simulink model "Sim"  (R2019b)
settings: Solver=VariableStepAuto  StartTime=0.0  StopTime=10.0  RelTol=1e-3
undefined symbols (not defined in the file): damping, DiscIntNeverNeededParam, Id0, inertia, initial_percentage, Iq0, J, K_damping, K_inertia, L_ap, L_inc, L_inc_inv, Ldd_inc, Ldq_inc, Lqq_inc, Psi_dm, Qp, Qx, R, Rs, Tob, Tsim, Ud0, Umd, Umq, Uq0, we0, weh
settings Model: SimulationMode=accelerator  Creator=Downstream  LastModifiedBy=Downstream

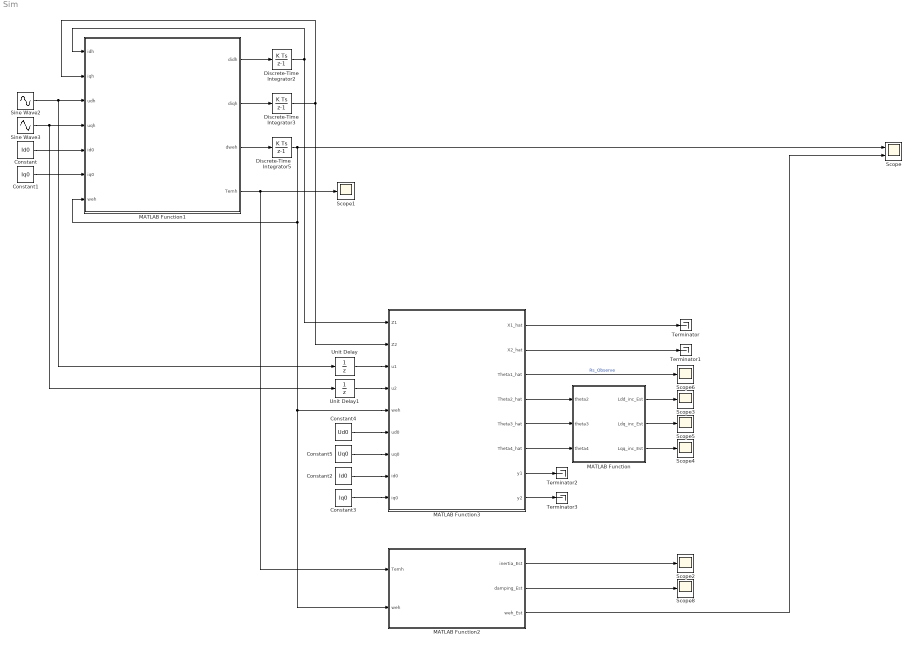
== system Sim ==
  Constant : Constant  Value=Id0  SampleTime=-1
  Constant1 : Constant  Value=Iq0  SampleTime=-1
  Constant2 : Constant  Value=Id0  SampleTime=-1
  Constant3 : Constant  Value=Iq0  SampleTime=-1
  Constant4 : Constant  Value=Ud0  SampleTime=-1
  Constant5 : Constant  Value=Uq0  SampleTime=-1
  Discrete-Time Integrator2 : DiscreteIntegrator  SampleTime=Tsim  ICPrevOutput=DiscIntNeverNeededParam  ICPrevScaledInput=DiscIntNeverNeededParam
  Discrete-Time Integrator3 : DiscreteIntegrator  SampleTime=Tsim  ICPrevOutput=DiscIntNeverNeededParam  ICPrevScaledInput=DiscIntNeverNeededParam
  Discrete-Time Integrator5 : DiscreteIntegrator  SampleTime=Tsim  ICPrevOutput=DiscIntNeverNeededParam  ICPrevScaledInput=DiscIntNeverNeededParam
  MATLAB Function : MATLAB Function  TreatAsAtomicUnit=on
  MATLAB Function1 : MATLAB Function  TreatAsAtomicUnit=on
  MATLAB Function2 : MATLAB Function  TreatAsAtomicUnit=on  SystemSampleTime=Tob
  MATLAB Function3 : MATLAB Function  TreatAsAtomicUnit=on  SystemSampleTime=Tob
  Scope : Scope  NumInputPorts=2
  Scope{1..6,8} (7 alike) : Scope
  Sine Wave2 : Sin  Amplitude=Umd  Frequency=weh  SampleTime=Tsim
  Sine Wave3 : Sin  Amplitude=Umq  Frequency=weh  Phase=pi/2  SampleTime=Tsim
  Terminator{,1..3} (4 alike) : Terminator
  Unit Delay : UnitDelay  SampleTime=Tob  HasFrameUpgradeWarning=on
  Unit Delay1 : UnitDelay  SampleTime=Tob  HasFrameUpgradeWarning=on
  wires:
  MATLAB Function1/1(didh) -> Discrete-Time Integrator2/1
  MATLAB Function1/2(diqh) -> Discrete-Time Integrator3/1
  Constant/1 -> MATLAB Function1/5(id0)
  Constant1/1 -> MATLAB Function1/6(iq0)
  MATLAB Function1/3(dweh) -> Discrete-Time Integrator5/1
  Constant2/1 -> MATLAB Function3/8(id0)
  Constant3/1 -> MATLAB Function3/9(iq0)
  Constant4/1 -> MATLAB Function3/6(ud0)
  Constant5/1 -> MATLAB Function3/7(uq0)
  MATLAB Function3/4(Theta2_hat) -> MATLAB Function/1(theta2)
  MATLAB Function3/5(Theta3_hat) -> MATLAB Function/2(theta3)
  MATLAB Function3/6(Theta4_hat) -> MATLAB Function/3(theta4)
  MATLAB Function/3(Lqq_inc_Est) -> Scope4/1
  MATLAB Function/2(Ldq_inc_Est) -> Scope5/1
  MATLAB Function/1(Ldd_inc_Est) -> Scope3/1
  MATLAB Function3/3(Theta1_hat) -> Scope6/1  "Rs_Observe"
  MATLAB Function2/3(weh_Est) -> Scope/2
  MATLAB Function2/1(inertia_Est) -> Scope2/1
  MATLAB Function2/2(damping_Est) -> Scope8/1
  Discrete-Time Integrator2/1 -> MATLAB Function3/1(Z1), MATLAB Function1/1(idh)
  Discrete-Time Integrator3/1 -> MATLAB Function3/2(Z2), MATLAB Function1/2(iqh)
  Sine Wave2/1 -> Unit Delay/1, MATLAB Function1/3(udh)
  Sine Wave3/1 -> Unit Delay1/1, MATLAB Function1/4(uqh)
  Discrete-Time Integrator5/1 -> MATLAB Function2/2(weh), MATLAB Function3/5(weh), MATLAB Function1/7(weh), Scope/1
  MATLAB Function1/4(Temh) -> MATLAB Function2/1(Temh), Scope1/1
  Unit Delay/1 -> MATLAB Function3/3(u1)
  Unit Delay1/1 -> MATLAB Function3/4(u2)
  MATLAB Function3/1(X1_hat) -> Terminator/1
  MATLAB Function3/2(X2_hat) -> Terminator1/1
  MATLAB Function3/7(y1) -> Terminator2/1
  MATLAB Function3/8(y2) -> Terminator3/1

== matlab function Sim/MATLAB Function1 ==
  data: idh input; didh output; iqh input; udh input; uqh input; id0 input; iq0 input; weh input; L_inc parameter; L_inc_inv parameter; L_ap parameter; we0 parameter; diqh output; inertia parameter; damping parameter; dweh output; Rs parameter; Psi_dm parameter; J parameter; Ldd_inc parameter; Ldq_inc parameter; Lqq_inc parameter; Temh output
function [didh,diqh,dweh,Temh] = PMSMSmallSignalModelANDFundamentalMode(idh,iqh,udh,uqh,id0,iq0,weh, L_inc, L_inc_inv, L_ap, we0, inertia, damping, Rs, Psi_dm, J, Ldd_inc, Ldq_inc, Lqq_inc)
ih = [idh;iqh];
uh = [udh;uqh];
Psi0 = L_ap * [id0;iq0] + [Psi_dm;0;];
dih = L_inc_inv * (uh - Rs * ih - we0 * J * L_inc * ih - weh * J * Psi0);
didh = dih(1,1);
diqh = dih(2,1);

P = 4; %pole pairs
Psi_d0 = Psi0(1,1);
Psi_q0 = Psi0(2,1);
Temh = 3/2 * P * ((Psi_d0 * iqh - Psi_q0 * idh) - Lqq_inc * id0 * iqh + Ldd_inc * iq0 * idh + Ldq_inc * (iqh * iq0 - idh * id0));
dweh = (Temh - damping * weh)/inertia;

== matlab function Sim/MATLAB Function ==
  data: theta2 input; Ldd_inc_Est output; Ldq_inc_Est output; theta3 input; theta4 input; Lqq_inc_Est output
function [Ldd_inc_Est, Ldq_inc_Est, Lqq_inc_Est] = L_inc_invANDSat(theta2,theta3,theta4)
L_inc_inv = [theta2, theta3; theta3  theta4];
L_inc = L_inc_inv ^ -1;
Ldd_inc_Est = L_inc(1,1);
Ldq_inc_Est = -L_inc(2,1);
Lqq_inc_Est = L_inc(2,2);

== matlab function Sim/MATLAB Function2 ==
  data: Temh input; inertia_Est output; weh input; damping_Est output; inertia parameter; damping parameter; Tob parameter; weh_Est output; K_inertia parameter; K_damping parameter; initial_percentage parameter
function [inertia_Est,damping_Est,weh_Est] = MechanicalOb(Temh,weh, inertia, damping, Tob, K_inertia, K_damping, initial_percentage)
persistent weh_hat inertia_hat damping_hat
if isempty(weh_hat)
    weh_hat = 0;
    inertia_hat = inertia * initial_percentage;
    damping_hat = damping * initial_percentage;
end
weh_tilde = weh_hat - weh;
weh_hat_dot = (1/inertia_hat) * (Temh - damping_hat * weh_hat);
weh_hat_nextpriod = weh_hat + weh_hat_dot * Tob;
inertia_hat = inertia_hat + Tob * K_inertia * weh_tilde * weh_hat_dot;
damping_hat = damping_hat + Tob * K_damping * weh_tilde * weh_hat;
weh_hat = weh_hat_nextpriod;
inertia_Est = inertia_hat;
damping_Est = damping_hat;
weh_Est = weh_hat;

== matlab function Sim/MATLAB Function3 ==
  data: Z1 input; X1_hat output; X2_hat output; Z2 input; u1 input; u2 input; weh input; ud0 input; uq0 input; id0 input; iq0 input; Tob parameter; Qp parameter; Qx parameter; R parameter; we0 parameter; Theta1_hat output; Theta2_hat output; Theta3_hat output; Theta4_hat output; y1 output; y2 output; L_inc_inv parameter; Rs parameter; initial_percentage parameter
function [X1_hat,X2_hat,Theta1_hat,Theta2_hat,Theta3_hat,Theta4_hat,y1,y2] = EKF_ParameterObserver(Z1,Z2,u1,u2, weh, ud0, uq0, id0, iq0 ,Tob,Qp,Qx,R,we0, L_inc_inv, Rs, initial_percentage)
persistent X_hat Theta_hat P_Theta_hat P_X_hat;
if isempty(X_hat)
    X_hat = [0;0];
end
if isempty(Theta_hat)
    Theta_hat = (1/initial_percentage) * [Rs;L_inc_inv(1,1);-L_inc_inv(2,1);L_inc_inv(2,2)] ;
    Theta_hat(1,1) = initial_percentage * Rs;
end
if isempty(P_Theta_hat)
    P_Theta_hat = zeros(4);
end
if isempty(P_X_hat)
    P_X_hat = zeros(2);
end

persistent difX_difTheta K_xk_1 difH_difTheta;
if isempty(difX_difTheta)
    difX_difTheta = zeros(2,4);
end
if isempty(K_xk_1)
    K_xk_1 = zeros(2,2);
end
if isempty(difH_difTheta)
    difH_difTheta = zeros(2,4);
end
U = [u1;u2];
Z = [Z1;Z2];
%Step1: Parameter Prioi Estimation
Theta_PE = Theta_hat;
P_Theta_PE = P_Theta_hat + Qp;
%Step2: State Prioi Estimation
Rs = Theta_PE(1,1) * eye(2);

% This J matrix definitation is in contrary with existing literature and
% the J in the ParamSetting.mlx file, this is because the DEKF observer
% first design is based on this definitation and will be correction to J =
% [0 -1; 1 0]; in the future work.
J = [0 1;-1 0;]; 



T = [Theta_PE(2,1),-Theta_PE(3,1);-Theta_PE(3,1),Theta_PE(4,1)];
A = (we0 * J - Rs * T);
%  Phi = eye(2) + A * Ts + 1/2 * A^2 * Ts^2 + 1/6 * A^3 * Ts^3;
Phi = eye(2) + Tob.*A;
% G = Ts *( eye(2) + 1/2 * A * Ts + 1/6 * A^2 * Ts^2);
G = Tob *( eye(2));
X_PE = Phi * X_hat + G * (U - weh/we0 * ([ud0;uq0;] - Theta_PE(1,1) * [id0;iq0;]));
P_X_PE = Phi * P_X_hat * Phi' + Qx;
%Step3: State Kalman Gain
K_xk = P_X_PE * T' * (T * P_X_PE * T' + R)^-1;
P_X_hat = (eye(2) - K_xk * T) * P_X_PE;
%Step4: Parameter Kalman Gain
difX_hat_difTheta = difX_difTheta - K_xk_1 * difH_difTheta;
difF_difTheta = -Tob .* [Theta_PE(2,1) *  X_hat(1) - Theta_PE(3,1) * X_hat(2),Theta_PE(1,1) * X_hat(1),-Theta_PE(1,1) * X_hat(2),0                         ;...
                       -Theta_PE(3,1) *  X_hat(1) + Theta_PE(4,1) * X_hat(2),0                       ,-Theta_PE(1,1) * X_hat(1),Theta_PE(1,1) * X_hat(2)  ;];
difF_difTheta = difF_difTheta + Phi * difX_hat_difTheta;
H_pk = [0,X_hat(1),-X_hat(2),0;0,0,-X_hat(1),X_hat(2)] + T * difF_difTheta;

K_pk = P_Theta_PE * H_pk' * (H_pk * P_Theta_PE * H_pk' + R)^-1;
P_Theta_hat = (eye(4) - K_pk * H_pk) * P_Theta_PE;
%Step5: State & Parameter Prediction
X_hat = X_PE + K_xk * (Z - T * X_PE);
Theta_hat = Theta_PE + K_pk * (Z - T * X_PE);
if(Theta_hat(1,1) > 1)
    Theta_hat(1,1) = 1;
elseif (Theta_hat(1,1) < 0)
    Theta_hat(1,1) = 0;
end
if(Theta_hat(2,1) > L_inc_inv(1,1)*100)
    Theta_hat(2,1) = L_inc_inv(1,1)*100;
elseif (Theta_hat(2,1) < L_inc_inv(1,1)/100)
    Theta_hat(2,1) = L_inc_inv(1,1)/100;
end
if(Theta_hat(3,1) <  -L_inc_inv(2,1)*100)
    Theta_hat(3,1) =   -L_inc_inv(2,1)*100;
elseif (Theta_hat(3,1) > -L_inc_inv(2,1)/100)
    Theta_hat(3,1) =   -L_inc_inv(2,1)/100;
end
if(Theta_hat(4,1) >  L_inc_inv(2,2)*100)
    Theta_hat(4,1) = L_inc_inv(2,2)*100;
elseif (Theta_hat(4,1) < L_inc_inv(2,2)/100)
    Theta_hat(4,1) = L_inc_inv(2,2)/100;
end
%Step6: Update the Parameter Kalman Gain
difX_difTheta = difF_difTheta;
K_xk_1 = K_xk;
difH_difTheta = H_pk;
X1_hat = X_hat(1,1);X2_hat = X_hat(2,1);
Theta1_hat = Theta_hat(1,1);Theta2_hat = Theta_hat(2,1);Theta3_hat = Theta_hat(3,1);Theta4_hat = Theta_hat(4,1);
Y = T * X_hat;
y1 = Y(1,1);
y2 = Y(2,1);
end
